simulink model "Powersystem_without_oscilloscopes"  (R2022b)
settings: Solver=ode45  StartTime=0.0  StopTime=25.000000  RelTol=1e-4  AbsTol=1e-5  EnableMultiTasking=on
undefined symbols (not defined in the file or in its folder): v_beta
libraries: simulink x11
(part 2 of 2)

== system Powersystem_without_oscilloscopes/Energylimits ==
  note: Power
  note: Energy
  Pref : Inport
  1-D Lookup Table : Lookup_n-D  NumberOfTableDimensions=1  BreakpointsForDimension1=[0,fracdemax,demax,1000*demax]  Table=[dpmax,dpmax,0,0]  InternalRulePriority=Speed  RndMeth=Simplest
  Constant : Constant  Value=dpmin
  Derivative : Derivative
  Integrator : Integrator
  delimit : Saturate  UpperLimit=demax  LowerLimit=demin
  tail control : simulink/Discontinuities/Saturation Dynamic  OutMin=[]  OutMax=[]  OutDataTypeStr=Inherit: Same as second input  OutDataType=sfix(16)  OutScaling=2^-10  DoSatur=off
  Pout : Outport
  wires:
  Integrator/1 -> delimit/1
  delimit/1 -> 1-D Lookup Table/1, Derivative/1
  Derivative/1 -> Pout/1
  1-D Lookup Table/1 -> tail control/1
  Constant/1 -> tail control/3
  Pref/1 -> tail control/2
  tail control/1 -> Integrator/1

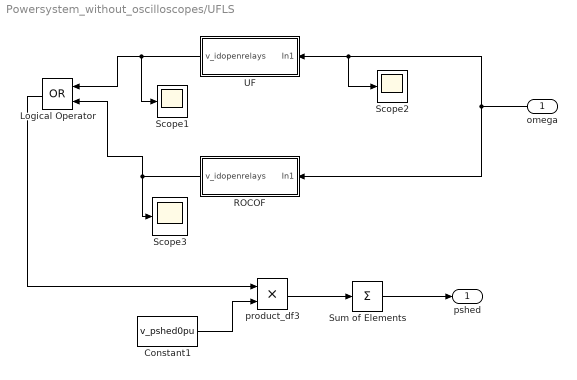
== system Powersystem_without_oscilloscopes/UFLS ==
  omega : Inport
  Constant1 : Constant  Value=v_pshed0pu
  Logical Operator : Logic  Operator=OR  AllPortsSameDT=off  OutDataTypeStr=boolean
  ROCOF : Subsystem
  Scope1 : Scope
  Scope2 : Scope
  Scope3 : Scope
  Sum of Elements : Sum  Inputs=+
  UF : Subsystem
  product_df3 : Product  RndMeth=Zero
  pshed : Outport
  wires:
  omega/1 -> Scope2/1, UF/1(In1), ROCOF/1(In1)
  UF/1(v_idopenrelays) -> Scope1/1, Logical Operator/1
  Sum of Elements/1 -> pshed/1
  Constant1/1 -> product_df3/2
  product_df3/1 -> Sum of Elements/1
  Logical Operator/1 -> product_df3/1
  ROCOF/1(v_idopenrelays) -> Scope3/1, Logical Operator/2

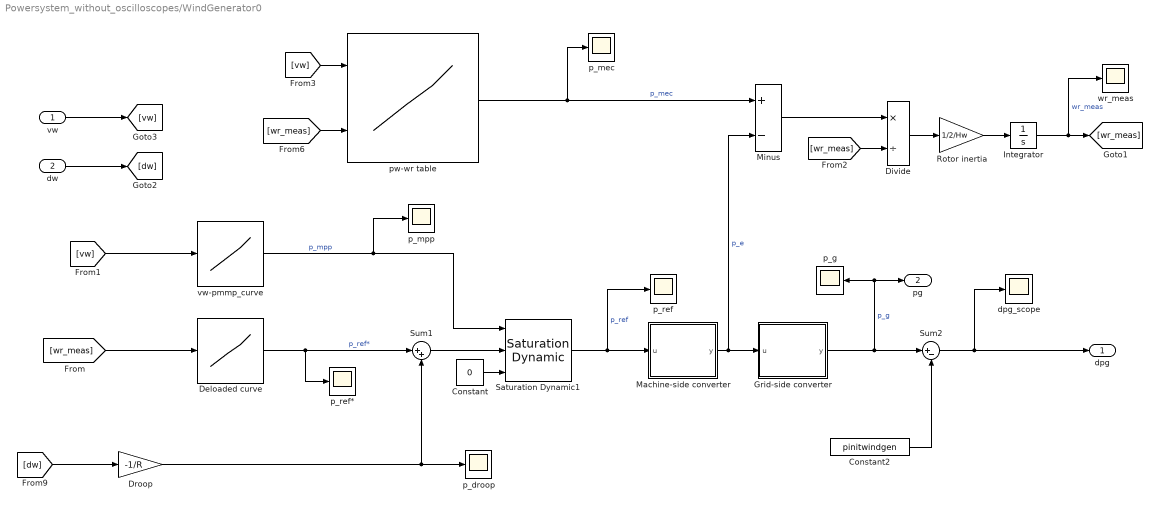
== system Powersystem_without_oscilloscopes/WindGenerator0 ==
  vw : Inport
  dw : Inport  Port=2
  Constant : Constant  Value=0
  Constant2 : Constant  Value=pinitwindgen
  Deloaded curve : Lookup_n-D  NumberOfTableDimensions=1  BreakpointsForDimension1=v_wrdel  Table=v_pwdel  InternalRulePriority=Speed  RndMeth=Simplest
  Divide : Product  Inputs=*/
  Droop : Gain  Gain=-1/R
  Grid-side converter : Subsystem  mask{T=Tc2, y0=pinitwindgen}
      mask prompts: T "Time constant (s)"; y0 "Initial condition (pu)"
  Integrator : Integrator  InitialCondition=wr0
  Machine-side converter : Subsystem  mask{T=Tc1, y0=pinitwindgen}
      mask prompts: T "Time constant (s)"; y0 "Initial condition (pu)"
  Minus : Sum  Inputs=+-
  Rotor inertia : Gain  Gain=1/2/Hw
  Saturation Dynamic1 : simulink/Discontinuities/Saturation Dynamic  OutMin=0  OutMax=[]  OutDataTypeStr=Inherit: Same as second input  OutDataType=fixdt(1, 16)  OutScaling=2^-10  DoSatur=off
  Sum1 : Sum  Inputs=|++
  Sum2 : Sum  Inputs=|+-
  dpg_scope : Scope
  p_droop : Scope
  p_g : Scope
  p_mec : Scope
  p_mpp : Scope
  p_ref : Scope
  p_ref* : Scope
  pw-wr table : Lookup_n-D  BreakpointsForDimension1=v_vw  BreakpointsForDimension2=v_wr  BreakpointsForDimension3=v_beta  Table=m_pw  InternalRulePriority=Speed  RndMeth=Simplest
      settings: InputPortMap=u0,u1
  vw-pmmp_curve : Lookup_n-D  NumberOfTableDimensions=1  BreakpointsForDimension1=v_vw  Table=v_pwmpp  InternalRulePriority=Speed  RndMeth=Simplest
  wr_meas : Scope
  dpg : Outport
  pg : Outport  Port=2
  wires:
  Sum2/1 -> dpg/1, dpg_scope/1
  [wr_meas] -> pw-wr table/2
  Deloaded curve/1 -> Sum1/1, p_ref*/1  "p_ref*"
  [dw] -> Droop/1
  Grid-side converter/1(y) -> Sum2/1, p_g/1, pg/1  "p_g"
  Saturation Dynamic1/1 -> p_ref/1, Machine-side converter/1(u)  "p_ref"
  [wr_meas] -> Deloaded curve/1
  Rotor inertia/1 -> Integrator/1
  [vw] -> pw-wr table/1
  pw-wr table/1 -> Minus/1, p_mec/1  "p_mec"
  Integrator/1 -> wr_meas/1, [wr_meas]  "wr_meas"
  vw/1 -> [vw]
  Sum1/1 -> Saturation Dynamic1/2
  Machine-side converter/1(y) -> Minus/2, Grid-side converter/1(u)  "p_e"
  vw-pmmp_curve/1 -> Saturation Dynamic1/1, p_mpp/1  "p_mpp"
  Constant2/1 -> Sum2/2
  dw/1 -> [dw]
  Constant/1 -> Saturation Dynamic1/3
  [vw] -> vw-pmmp_curve/1
  Droop/1 -> p_droop/1, Sum1/2
  Minus/1 -> Divide/1
  Divide/1 -> Rotor inertia/1
  [wr_meas] -> Divide/2

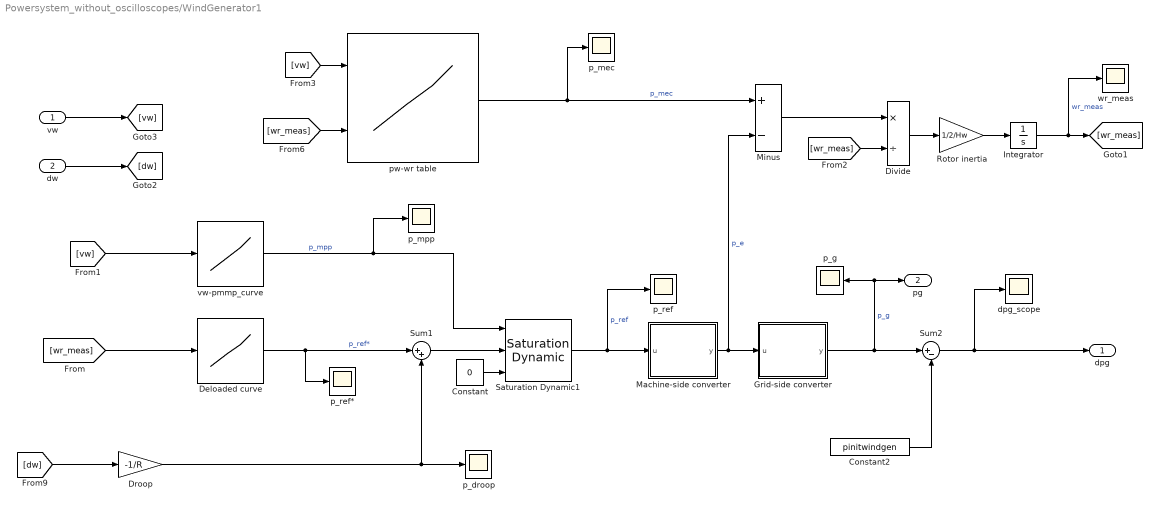
== system Powersystem_without_oscilloscopes/WindGenerator1 ==
  vw : Inport
  dw : Inport  Port=2
  Constant : Constant  Value=0
  Constant2 : Constant  Value=pinitwindgen
  Deloaded curve : Lookup_n-D  NumberOfTableDimensions=1  BreakpointsForDimension1=v_wrdel  Table=v_pwdel  InternalRulePriority=Speed  RndMeth=Simplest
  Divide : Product  Inputs=*/
  Droop : Gain  Gain=-1/R
  Grid-side converter : Subsystem  mask{T=Tc2, y0=pinitwindgen}
      mask prompts: T "Time constant (s)"; y0 "Initial condition (pu)"
  Integrator : Integrator  InitialCondition=wr0
  Machine-side converter : Subsystem  mask{T=Tc1, y0=pinitwindgen}
      mask prompts: T "Time constant (s)"; y0 "Initial condition (pu)"
  Minus : Sum  Inputs=+-
  Rotor inertia : Gain  Gain=1/2/Hw
  Saturation Dynamic1 : simulink/Discontinuities/Saturation Dynamic  OutMin=0  OutMax=[]  OutDataTypeStr=Inherit: Same as second input  OutDataType=fixdt(1, 16)  OutScaling=2^-10  DoSatur=off
  Sum1 : Sum  Inputs=|++
  Sum2 : Sum  Inputs=|+-
  dpg_scope : Scope
  p_droop : Scope
  p_g : Scope
  p_mec : Scope
  p_mpp : Scope
  p_ref : Scope
  p_ref* : Scope
  pw-wr table : Lookup_n-D  BreakpointsForDimension1=v_vw  BreakpointsForDimension2=v_wr  BreakpointsForDimension3=v_beta  Table=m_pw  InternalRulePriority=Speed  RndMeth=Simplest
      settings: InputPortMap=u0,u1
  vw-pmmp_curve : Lookup_n-D  NumberOfTableDimensions=1  BreakpointsForDimension1=v_vw  Table=v_pwmpp  InternalRulePriority=Speed  RndMeth=Simplest
  wr_meas : Scope
  dpg : Outport
  pg : Outport  Port=2
  wires:
  Sum2/1 -> dpg/1, dpg_scope/1
  [wr_meas] -> pw-wr table/2
  Deloaded curve/1 -> Sum1/1, p_ref*/1  "p_ref*"
  [dw] -> Droop/1
  Grid-side converter/1(y) -> Sum2/1, p_g/1, pg/1  "p_g"
  Saturation Dynamic1/1 -> p_ref/1, Machine-side converter/1(u)  "p_ref"
  [wr_meas] -> Deloaded curve/1
  Rotor inertia/1 -> Integrator/1
  [vw] -> pw-wr table/1
  pw-wr table/1 -> Minus/1, p_mec/1  "p_mec"
  Integrator/1 -> wr_meas/1, [wr_meas]  "wr_meas"
  vw/1 -> [vw]
  Sum1/1 -> Saturation Dynamic1/2
  Machine-side converter/1(y) -> Minus/2, Grid-side converter/1(u)  "p_e"
  vw-pmmp_curve/1 -> Saturation Dynamic1/1, p_mpp/1  "p_mpp"
  Constant2/1 -> Sum2/2
  dw/1 -> [dw]
  Constant/1 -> Saturation Dynamic1/3
  [vw] -> vw-pmmp_curve/1
  Droop/1 -> p_droop/1, Sum1/2
  Minus/1 -> Divide/1
  Divide/1 -> Rotor inertia/1
  [wr_meas] -> Divide/2

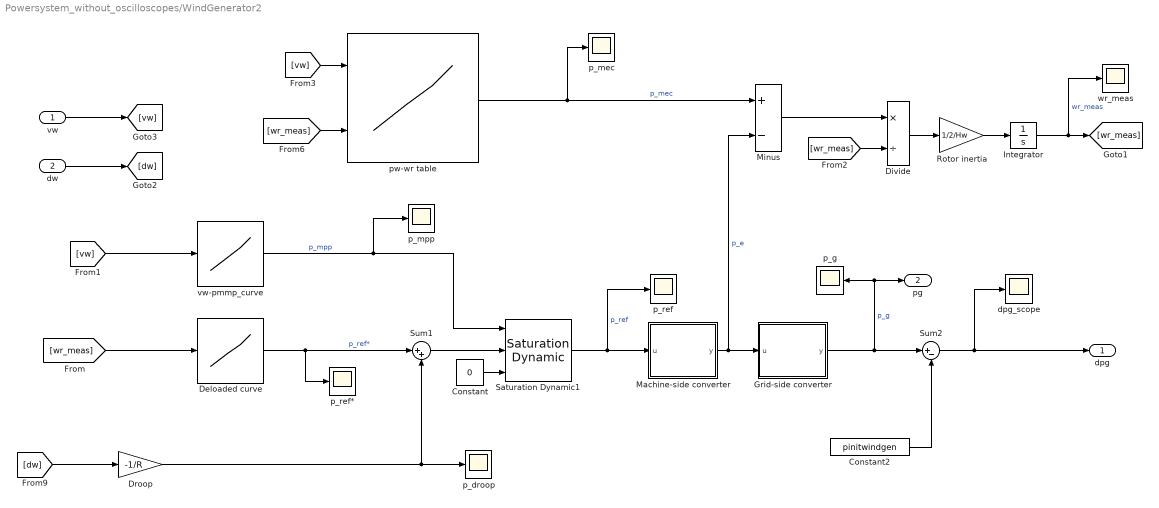
== system Powersystem_without_oscilloscopes/WindGenerator2 ==
  vw : Inport
  dw : Inport  Port=2
  Constant : Constant  Value=0
  Constant2 : Constant  Value=pinitwindgen
  Deloaded curve : Lookup_n-D  NumberOfTableDimensions=1  BreakpointsForDimension1=v_wrdel  Table=v_pwdel  InternalRulePriority=Speed  RndMeth=Simplest
  Divide : Product  Inputs=*/
  Droop : Gain  Gain=-1/R
  Grid-side converter : Subsystem  mask{T=Tc2, y0=pinitwindgen}
      mask prompts: T "Time constant (s)"; y0 "Initial condition (pu)"
  Integrator : Integrator  InitialCondition=wr0
  Machine-side converter : Subsystem  mask{T=Tc1, y0=pinitwindgen}
      mask prompts: T "Time constant (s)"; y0 "Initial condition (pu)"
  Minus : Sum  Inputs=+-
  Rotor inertia : Gain  Gain=1/2/Hw
  Saturation Dynamic1 : simulink/Discontinuities/Saturation Dynamic  OutMin=0  OutMax=[]  OutDataTypeStr=Inherit: Same as second input  OutDataType=fixdt(1, 16)  OutScaling=2^-10  DoSatur=off
  Sum1 : Sum  Inputs=|++
  Sum2 : Sum  Inputs=|+-
  dpg_scope : Scope
  p_droop : Scope
  p_g : Scope
  p_mec : Scope
  p_mpp : Scope
  p_ref : Scope
  p_ref* : Scope
  pw-wr table : Lookup_n-D  BreakpointsForDimension1=v_vw  BreakpointsForDimension2=v_wr  BreakpointsForDimension3=v_beta  Table=m_pw  InternalRulePriority=Speed  RndMeth=Simplest
      settings: InputPortMap=u0,u1
  vw-pmmp_curve : Lookup_n-D  NumberOfTableDimensions=1  BreakpointsForDimension1=v_vw  Table=v_pwmpp  InternalRulePriority=Speed  RndMeth=Simplest
  wr_meas : Scope
  dpg : Outport
  pg : Outport  Port=2
  wires:
  Sum2/1 -> dpg/1, dpg_scope/1
  [wr_meas] -> pw-wr table/2
  Deloaded curve/1 -> Sum1/1, p_ref*/1  "p_ref*"
  [dw] -> Droop/1
  Grid-side converter/1(y) -> Sum2/1, p_g/1, pg/1  "p_g"
  Saturation Dynamic1/1 -> p_ref/1, Machine-side converter/1(u)  "p_ref"
  [wr_meas] -> Deloaded curve/1
  Rotor inertia/1 -> Integrator/1
  [vw] -> pw-wr table/1
  pw-wr table/1 -> Minus/1, p_mec/1  "p_mec"
  Integrator/1 -> wr_meas/1, [wr_meas]  "wr_meas"
  vw/1 -> [vw]
  Sum1/1 -> Saturation Dynamic1/2
  Machine-side converter/1(y) -> Minus/2, Grid-side converter/1(u)  "p_e"
  vw-pmmp_curve/1 -> Saturation Dynamic1/1, p_mpp/1  "p_mpp"
  Constant2/1 -> Sum2/2
  dw/1 -> [dw]
  Constant/1 -> Saturation Dynamic1/3
  [vw] -> vw-pmmp_curve/1
  Droop/1 -> p_droop/1, Sum1/2
  Minus/1 -> Divide/1
  Divide/1 -> Rotor inertia/1
  [wr_meas] -> Divide/2

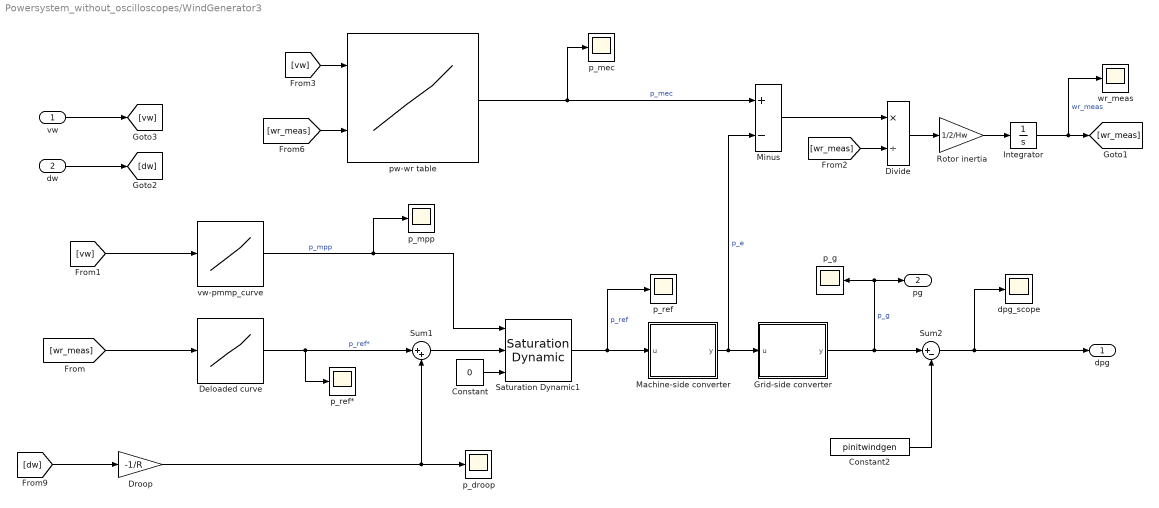
== system Powersystem_without_oscilloscopes/WindGenerator3 ==
  vw : Inport
  dw : Inport  Port=2
  Constant : Constant  Value=0
  Constant2 : Constant  Value=pinitwindgen
  Deloaded curve : Lookup_n-D  NumberOfTableDimensions=1  BreakpointsForDimension1=v_wrdel  Table=v_pwdel  InternalRulePriority=Speed  RndMeth=Simplest
  Divide : Product  Inputs=*/
  Droop : Gain  Gain=-1/R
  Grid-side converter : Subsystem  mask{T=Tc2, y0=pinitwindgen}
      mask prompts: T "Time constant (s)"; y0 "Initial condition (pu)"
  Integrator : Integrator  InitialCondition=wr0
  Machine-side converter : Subsystem  mask{T=Tc1, y0=pinitwindgen}
      mask prompts: T "Time constant (s)"; y0 "Initial condition (pu)"
  Minus : Sum  Inputs=+-
  Rotor inertia : Gain  Gain=1/2/Hw
  Saturation Dynamic1 : simulink/Discontinuities/Saturation Dynamic  OutMin=0  OutMax=[]  OutDataTypeStr=Inherit: Same as second input  OutDataType=fixdt(1, 16)  OutScaling=2^-10  DoSatur=off
  Sum1 : Sum  Inputs=|++
  Sum2 : Sum  Inputs=|+-
  dpg_scope : Scope
  p_droop : Scope
  p_g : Scope
  p_mec : Scope
  p_mpp : Scope
  p_ref : Scope
  p_ref* : Scope
  pw-wr table : Lookup_n-D  BreakpointsForDimension1=v_vw  BreakpointsForDimension2=v_wr  BreakpointsForDimension3=v_beta  Table=m_pw  InternalRulePriority=Speed  RndMeth=Simplest
      settings: InputPortMap=u0,u1
  vw-pmmp_curve : Lookup_n-D  NumberOfTableDimensions=1  BreakpointsForDimension1=v_vw  Table=v_pwmpp  InternalRulePriority=Speed  RndMeth=Simplest
  wr_meas : Scope
  dpg : Outport
  pg : Outport  Port=2
  wires:
  Sum2/1 -> dpg/1, dpg_scope/1
  [wr_meas] -> pw-wr table/2
  Deloaded curve/1 -> Sum1/1, p_ref*/1  "p_ref*"
  [dw] -> Droop/1
  Grid-side converter/1(y) -> Sum2/1, p_g/1, pg/1  "p_g"
  Saturation Dynamic1/1 -> p_ref/1, Machine-side converter/1(u)  "p_ref"
  [wr_meas] -> Deloaded curve/1
  Rotor inertia/1 -> Integrator/1
  [vw] -> pw-wr table/1
  pw-wr table/1 -> Minus/1, p_mec/1  "p_mec"
  Integrator/1 -> wr_meas/1, [wr_meas]  "wr_meas"
  vw/1 -> [vw]
  Sum1/1 -> Saturation Dynamic1/2
  Machine-side converter/1(y) -> Minus/2, Grid-side converter/1(u)  "p_e"
  vw-pmmp_curve/1 -> Saturation Dynamic1/1, p_mpp/1  "p_mpp"
  Constant2/1 -> Sum2/2
  dw/1 -> [dw]
  Constant/1 -> Saturation Dynamic1/3
  [vw] -> vw-pmmp_curve/1
  Droop/1 -> p_droop/1, Sum1/2
  Minus/1 -> Divide/1
  Divide/1 -> Rotor inertia/1
  [wr_meas] -> Divide/2

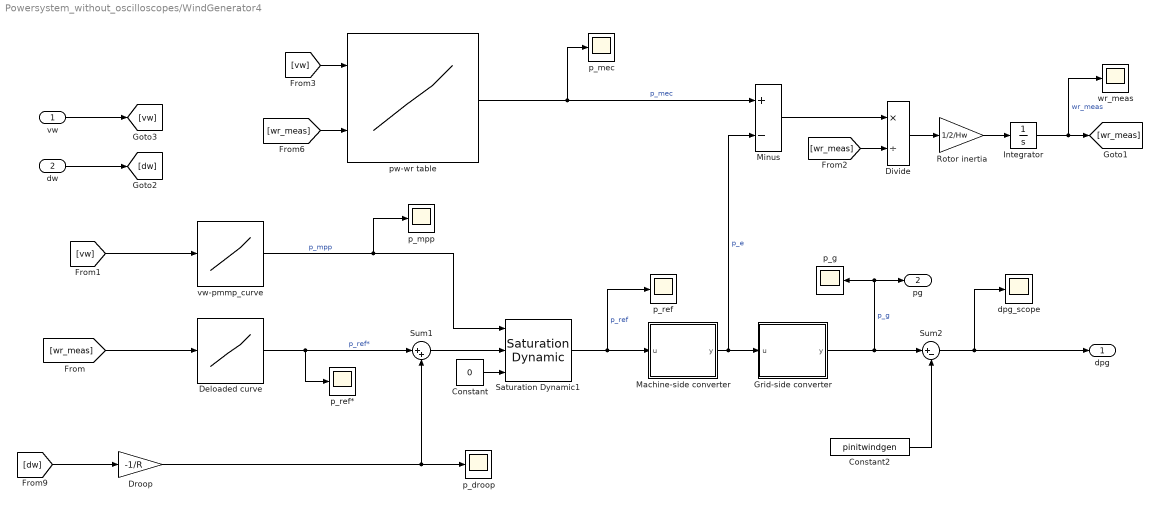
== system Powersystem_without_oscilloscopes/WindGenerator4 ==
  vw : Inport
  dw : Inport  Port=2
  Constant : Constant  Value=0
  Constant2 : Constant  Value=pinitwindgen
  Deloaded curve : Lookup_n-D  NumberOfTableDimensions=1  BreakpointsForDimension1=v_wrdel  Table=v_pwdel  InternalRulePriority=Speed  RndMeth=Simplest
  Divide : Product  Inputs=*/
  Droop : Gain  Gain=-1/R
  Grid-side converter : Subsystem  mask{T=Tc2, y0=pinitwindgen}
      mask prompts: T "Time constant (s)"; y0 "Initial condition (pu)"
  Integrator : Integrator  InitialCondition=wr0
  Machine-side converter : Subsystem  mask{T=Tc1, y0=pinitwindgen}
      mask prompts: T "Time constant (s)"; y0 "Initial condition (pu)"
  Minus : Sum  Inputs=+-
  Rotor inertia : Gain  Gain=1/2/Hw
  Saturation Dynamic1 : simulink/Discontinuities/Saturation Dynamic  OutMin=0  OutMax=[]  OutDataTypeStr=Inherit: Same as second input  OutDataType=fixdt(1, 16)  OutScaling=2^-10  DoSatur=off
  Sum1 : Sum  Inputs=|++
  Sum2 : Sum  Inputs=|+-
  dpg_scope : Scope
  p_droop : Scope
  p_g : Scope
  p_mec : Scope
  p_mpp : Scope
  p_ref : Scope
  p_ref* : Scope
  pw-wr table : Lookup_n-D  BreakpointsForDimension1=v_vw  BreakpointsForDimension2=v_wr  BreakpointsForDimension3=v_beta  Table=m_pw  InternalRulePriority=Speed  RndMeth=Simplest
      settings: InputPortMap=u0,u1
  vw-pmmp_curve : Lookup_n-D  NumberOfTableDimensions=1  BreakpointsForDimension1=v_vw  Table=v_pwmpp  InternalRulePriority=Speed  RndMeth=Simplest
  wr_meas : Scope
  dpg : Outport
  pg : Outport  Port=2
  wires:
  Sum2/1 -> dpg/1, dpg_scope/1
  [wr_meas] -> pw-wr table/2
  Deloaded curve/1 -> Sum1/1, p_ref*/1  "p_ref*"
  [dw] -> Droop/1
  Grid-side converter/1(y) -> Sum2/1, p_g/1, pg/1  "p_g"
  Saturation Dynamic1/1 -> p_ref/1, Machine-side converter/1(u)  "p_ref"
  [wr_meas] -> Deloaded curve/1
  Rotor inertia/1 -> Integrator/1
  [vw] -> pw-wr table/1
  pw-wr table/1 -> Minus/1, p_mec/1  "p_mec"
  Integrator/1 -> wr_meas/1, [wr_meas]  "wr_meas"
  vw/1 -> [vw]
  Sum1/1 -> Saturation Dynamic1/2
  Machine-side converter/1(y) -> Minus/2, Grid-side converter/1(u)  "p_e"
  vw-pmmp_curve/1 -> Saturation Dynamic1/1, p_mpp/1  "p_mpp"
  Constant2/1 -> Sum2/2
  dw/1 -> [dw]
  Constant/1 -> Saturation Dynamic1/3
  [vw] -> vw-pmmp_curve/1
  Droop/1 -> p_droop/1, Sum1/2
  Minus/1 -> Divide/1
  Divide/1 -> Rotor inertia/1
  [wr_meas] -> Divide/2

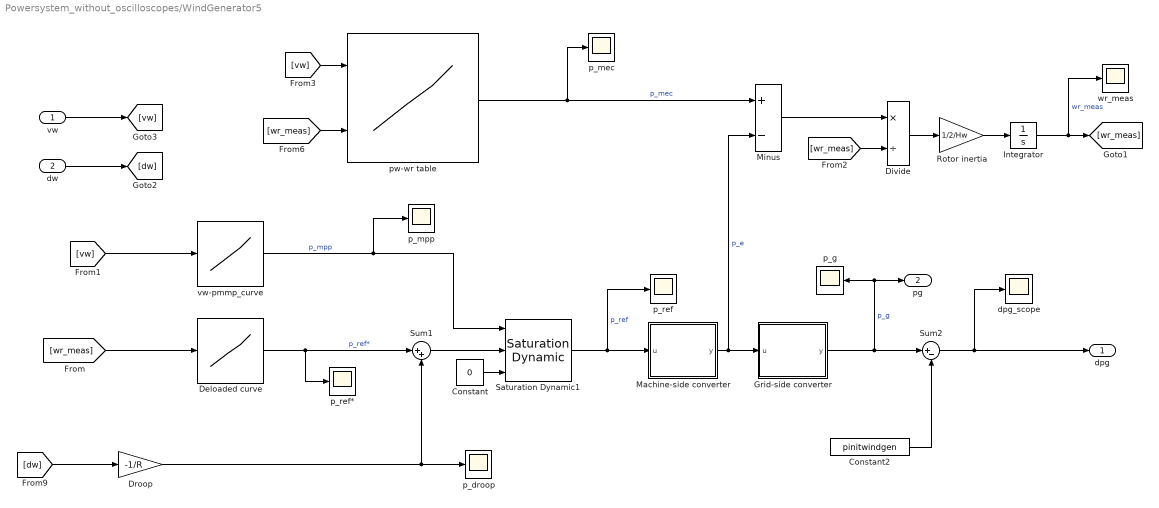
== system Powersystem_without_oscilloscopes/WindGenerator5 ==
  vw : Inport
  dw : Inport  Port=2
  Constant : Constant  Value=0
  Constant2 : Constant  Value=pinitwindgen
  Deloaded curve : Lookup_n-D  NumberOfTableDimensions=1  BreakpointsForDimension1=v_wrdel  Table=v_pwdel  InternalRulePriority=Speed  RndMeth=Simplest
  Divide : Product  Inputs=*/
  Droop : Gain  Gain=-1/R
  Grid-side converter : Subsystem  mask{T=Tc2, y0=pinitwindgen}
      mask prompts: T "Time constant (s)"; y0 "Initial condition (pu)"
  Integrator : Integrator  InitialCondition=wr0
  Machine-side converter : Subsystem  mask{T=Tc1, y0=pinitwindgen}
      mask prompts: T "Time constant (s)"; y0 "Initial condition (pu)"
  Minus : Sum  Inputs=+-
  Rotor inertia : Gain  Gain=1/2/Hw
  Saturation Dynamic1 : simulink/Discontinuities/Saturation Dynamic  OutMin=0  OutMax=[]  OutDataTypeStr=Inherit: Same as second input  OutDataType=fixdt(1, 16)  OutScaling=2^-10  DoSatur=off
  Sum1 : Sum  Inputs=|++
  Sum2 : Sum  Inputs=|+-
  dpg_scope : Scope
  p_droop : Scope
  p_g : Scope
  p_mec : Scope
  p_mpp : Scope
  p_ref : Scope
  p_ref* : Scope
  pw-wr table : Lookup_n-D  BreakpointsForDimension1=v_vw  BreakpointsForDimension2=v_wr  BreakpointsForDimension3=v_beta  Table=m_pw  InternalRulePriority=Speed  RndMeth=Simplest
      settings: InputPortMap=u0,u1
  vw-pmmp_curve : Lookup_n-D  NumberOfTableDimensions=1  BreakpointsForDimension1=v_vw  Table=v_pwmpp  InternalRulePriority=Speed  RndMeth=Simplest
  wr_meas : Scope
  dpg : Outport
  pg : Outport  Port=2
  wires:
  Sum2/1 -> dpg/1, dpg_scope/1
  [wr_meas] -> pw-wr table/2
  Deloaded curve/1 -> Sum1/1, p_ref*/1  "p_ref*"
  [dw] -> Droop/1
  Grid-side converter/1(y) -> Sum2/1, p_g/1, pg/1  "p_g"
  Saturation Dynamic1/1 -> p_ref/1, Machine-side converter/1(u)  "p_ref"
  [wr_meas] -> Deloaded curve/1
  Rotor inertia/1 -> Integrator/1
  [vw] -> pw-wr table/1
  pw-wr table/1 -> Minus/1, p_mec/1  "p_mec"
  Integrator/1 -> wr_meas/1, [wr_meas]  "wr_meas"
  vw/1 -> [vw]
  Sum1/1 -> Saturation Dynamic1/2
  Machine-side converter/1(y) -> Minus/2, Grid-side converter/1(u)  "p_e"
  vw-pmmp_curve/1 -> Saturation Dynamic1/1, p_mpp/1  "p_mpp"
  Constant2/1 -> Sum2/2
  dw/1 -> [dw]
  Constant/1 -> Saturation Dynamic1/3
  [vw] -> vw-pmmp_curve/1
  Droop/1 -> p_droop/1, Sum1/2
  Minus/1 -> Divide/1
  Divide/1 -> Rotor inertia/1
  [wr_meas] -> Divide/2

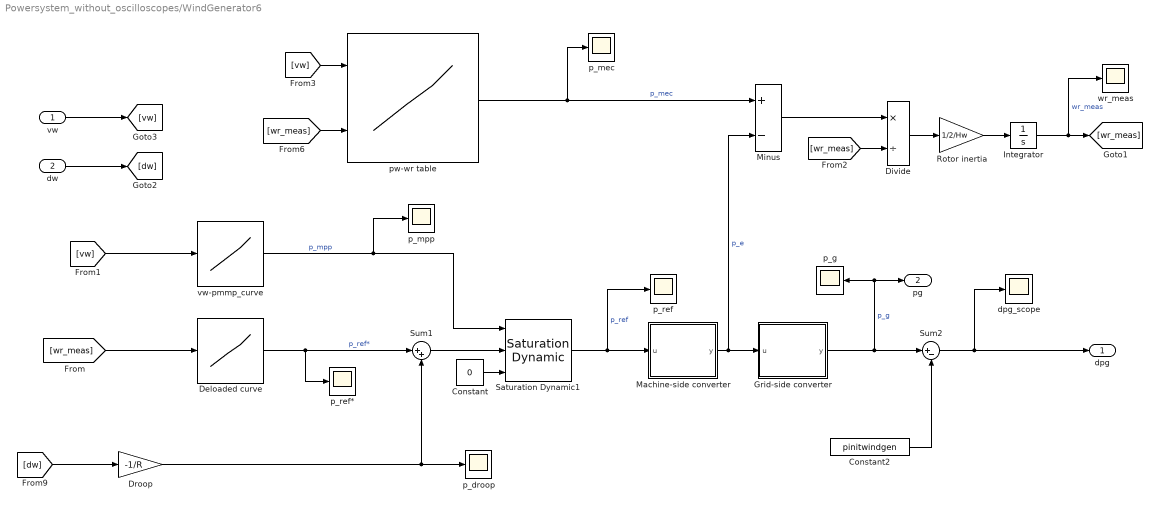
== system Powersystem_without_oscilloscopes/WindGenerator6 ==
  vw : Inport
  dw : Inport  Port=2
  Constant : Constant  Value=0
  Constant2 : Constant  Value=pinitwindgen
  Deloaded curve : Lookup_n-D  NumberOfTableDimensions=1  BreakpointsForDimension1=v_wrdel  Table=v_pwdel  InternalRulePriority=Speed  RndMeth=Simplest
  Divide : Product  Inputs=*/
  Droop : Gain  Gain=-1/R
  Grid-side converter : Subsystem  mask{T=Tc2, y0=pinitwindgen}
      mask prompts: T "Time constant (s)"; y0 "Initial condition (pu)"
  Integrator : Integrator  InitialCondition=wr0
  Machine-side converter : Subsystem  mask{T=Tc1, y0=pinitwindgen}
      mask prompts: T "Time constant (s)"; y0 "Initial condition (pu)"
  Minus : Sum  Inputs=+-
  Rotor inertia : Gain  Gain=1/2/Hw
  Saturation Dynamic1 : simulink/Discontinuities/Saturation Dynamic  OutMin=0  OutMax=[]  OutDataTypeStr=Inherit: Same as second input  OutDataType=fixdt(1, 16)  OutScaling=2^-10  DoSatur=off
  Sum1 : Sum  Inputs=|++
  Sum2 : Sum  Inputs=|+-
  dpg_scope : Scope
  p_droop : Scope
  p_g : Scope
  p_mec : Scope
  p_mpp : Scope
  p_ref : Scope
  p_ref* : Scope
  pw-wr table : Lookup_n-D  BreakpointsForDimension1=v_vw  BreakpointsForDimension2=v_wr  BreakpointsForDimension3=v_beta  Table=m_pw  InternalRulePriority=Speed  RndMeth=Simplest
      settings: InputPortMap=u0,u1
  vw-pmmp_curve : Lookup_n-D  NumberOfTableDimensions=1  BreakpointsForDimension1=v_vw  Table=v_pwmpp  InternalRulePriority=Speed  RndMeth=Simplest
  wr_meas : Scope
  dpg : Outport
  pg : Outport  Port=2
  wires:
  Sum2/1 -> dpg/1, dpg_scope/1
  [wr_meas] -> pw-wr table/2
  Deloaded curve/1 -> Sum1/1, p_ref*/1  "p_ref*"
  [dw] -> Droop/1
  Grid-side converter/1(y) -> Sum2/1, p_g/1, pg/1  "p_g"
  Saturation Dynamic1/1 -> p_ref/1, Machine-side converter/1(u)  "p_ref"
  [wr_meas] -> Deloaded curve/1
  Rotor inertia/1 -> Integrator/1
  [vw] -> pw-wr table/1
  pw-wr table/1 -> Minus/1, p_mec/1  "p_mec"
  Integrator/1 -> wr_meas/1, [wr_meas]  "wr_meas"
  vw/1 -> [vw]
  Sum1/1 -> Saturation Dynamic1/2
  Machine-side converter/1(y) -> Minus/2, Grid-side converter/1(u)  "p_e"
  vw-pmmp_curve/1 -> Saturation Dynamic1/1, p_mpp/1  "p_mpp"
  Constant2/1 -> Sum2/2
  dw/1 -> [dw]
  Constant/1 -> Saturation Dynamic1/3
  [vw] -> vw-pmmp_curve/1
  Droop/1 -> p_droop/1, Sum1/2
  Minus/1 -> Divide/1
  Divide/1 -> Rotor inertia/1
  [wr_meas] -> Divide/2

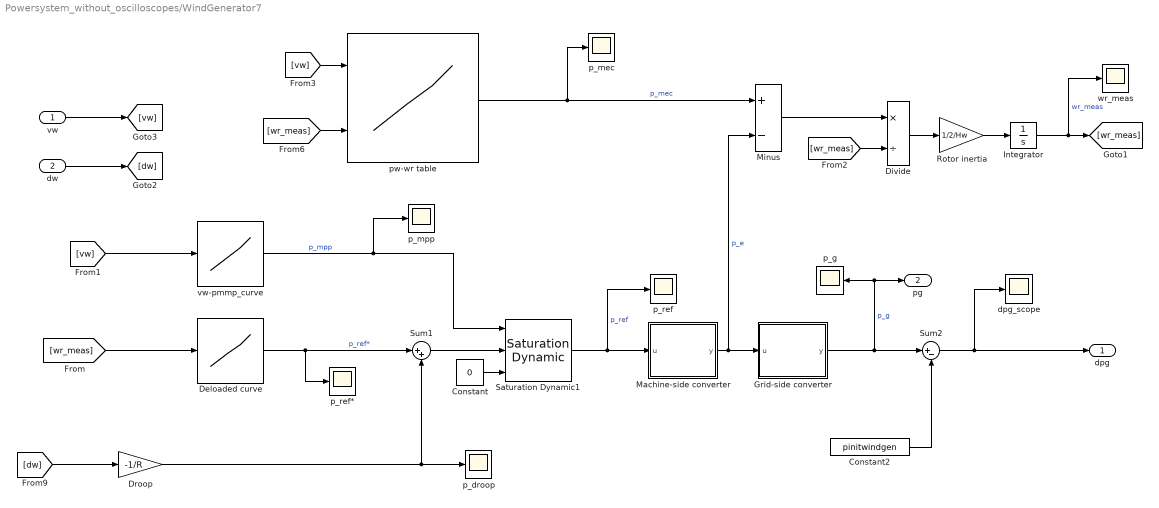
== system Powersystem_without_oscilloscopes/WindGenerator7 ==
  vw : Inport
  dw : Inport  Port=2
  Constant : Constant  Value=0
  Constant2 : Constant  Value=pinitwindgen
  Deloaded curve : Lookup_n-D  NumberOfTableDimensions=1  BreakpointsForDimension1=v_wrdel  Table=v_pwdel  InternalRulePriority=Speed  RndMeth=Simplest
  Divide : Product  Inputs=*/
  Droop : Gain  Gain=-1/R
  Grid-side converter : Subsystem  mask{T=Tc2, y0=pinitwindgen}
      mask prompts: T "Time constant (s)"; y0 "Initial condition (pu)"
  Integrator : Integrator  InitialCondition=wr0
  Machine-side converter : Subsystem  mask{T=Tc1, y0=pinitwindgen}
      mask prompts: T "Time constant (s)"; y0 "Initial condition (pu)"
  Minus : Sum  Inputs=+-
  Rotor inertia : Gain  Gain=1/2/Hw
  Saturation Dynamic1 : simulink/Discontinuities/Saturation Dynamic  OutMin=0  OutMax=[]  OutDataTypeStr=Inherit: Same as second input  OutDataType=fixdt(1, 16)  OutScaling=2^-10  DoSatur=off
  Sum1 : Sum  Inputs=|++
  Sum2 : Sum  Inputs=|+-
  dpg_scope : Scope
  p_droop : Scope
  p_g : Scope
  p_mec : Scope
  p_mpp : Scope
  p_ref : Scope
  p_ref* : Scope
  pw-wr table : Lookup_n-D  BreakpointsForDimension1=v_vw  BreakpointsForDimension2=v_wr  BreakpointsForDimension3=v_beta  Table=m_pw  InternalRulePriority=Speed  RndMeth=Simplest
      settings: InputPortMap=u0,u1
  vw-pmmp_curve : Lookup_n-D  NumberOfTableDimensions=1  BreakpointsForDimension1=v_vw  Table=v_pwmpp  InternalRulePriority=Speed  RndMeth=Simplest
  wr_meas : Scope
  dpg : Outport
  pg : Outport  Port=2
  wires:
  Sum2/1 -> dpg/1, dpg_scope/1
  [wr_meas] -> pw-wr table/2
  Deloaded curve/1 -> Sum1/1, p_ref*/1  "p_ref*"
  [dw] -> Droop/1
  Grid-side converter/1(y) -> Sum2/1, p_g/1, pg/1  "p_g"
  Saturation Dynamic1/1 -> p_ref/1, Machine-side converter/1(u)  "p_ref"
  [wr_meas] -> Deloaded curve/1
  Rotor inertia/1 -> Integrator/1
  [vw] -> pw-wr table/1
  pw-wr table/1 -> Minus/1, p_mec/1  "p_mec"
  Integrator/1 -> wr_meas/1, [wr_meas]  "wr_meas"
  vw/1 -> [vw]
  Sum1/1 -> Saturation Dynamic1/2
  Machine-side converter/1(y) -> Minus/2, Grid-side converter/1(u)  "p_e"
  vw-pmmp_curve/1 -> Saturation Dynamic1/1, p_mpp/1  "p_mpp"
  Constant2/1 -> Sum2/2
  dw/1 -> [dw]
  Constant/1 -> Saturation Dynamic1/3
  [vw] -> vw-pmmp_curve/1
  Droop/1 -> p_droop/1, Sum1/2
  Minus/1 -> Divide/1
  Divide/1 -> Rotor inertia/1
  [wr_meas] -> Divide/2

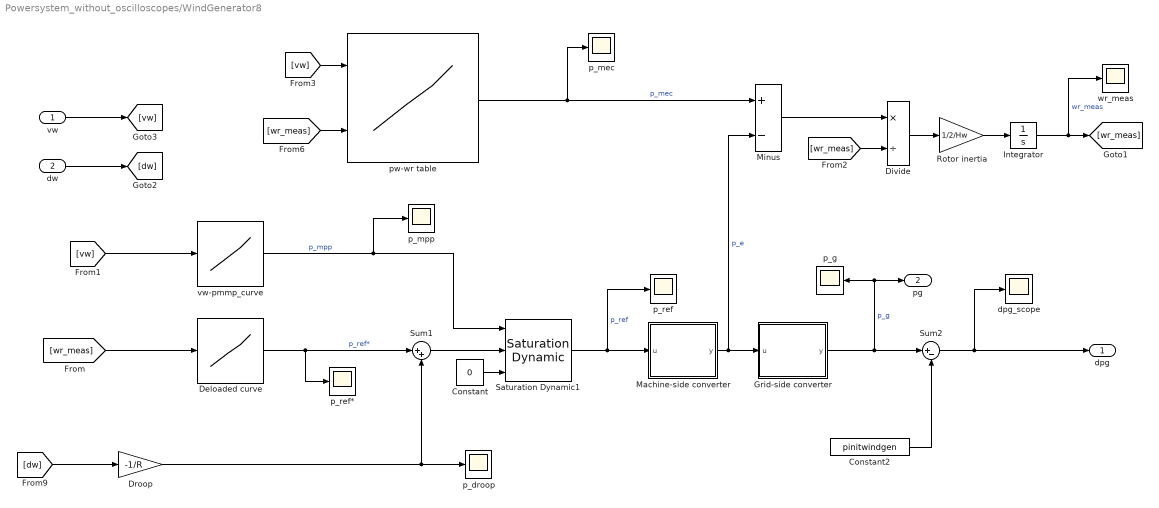
== system Powersystem_without_oscilloscopes/WindGenerator8 ==
  vw : Inport
  dw : Inport  Port=2
  Constant : Constant  Value=0
  Constant2 : Constant  Value=pinitwindgen
  Deloaded curve : Lookup_n-D  NumberOfTableDimensions=1  BreakpointsForDimension1=v_wrdel  Table=v_pwdel  InternalRulePriority=Speed  RndMeth=Simplest
  Divide : Product  Inputs=*/
  Droop : Gain  Gain=-1/R
  Grid-side converter : Subsystem  mask{T=Tc2, y0=pinitwindgen}
      mask prompts: T "Time constant (s)"; y0 "Initial condition (pu)"
  Integrator : Integrator  InitialCondition=wr0
  Machine-side converter : Subsystem  mask{T=Tc1, y0=pinitwindgen}
      mask prompts: T "Time constant (s)"; y0 "Initial condition (pu)"
  Minus : Sum  Inputs=+-
  Rotor inertia : Gain  Gain=1/2/Hw
  Saturation Dynamic1 : simulink/Discontinuities/Saturation Dynamic  OutMin=0  OutMax=[]  OutDataTypeStr=Inherit: Same as second input  OutDataType=fixdt(1, 16)  OutScaling=2^-10  DoSatur=off
  Sum1 : Sum  Inputs=|++
  Sum2 : Sum  Inputs=|+-
  dpg_scope : Scope
  p_droop : Scope
  p_g : Scope
  p_mec : Scope
  p_mpp : Scope
  p_ref : Scope
  p_ref* : Scope
  pw-wr table : Lookup_n-D  BreakpointsForDimension1=v_vw  BreakpointsForDimension2=v_wr  BreakpointsForDimension3=v_beta  Table=m_pw  InternalRulePriority=Speed  RndMeth=Simplest
      settings: InputPortMap=u0,u1
  vw-pmmp_curve : Lookup_n-D  NumberOfTableDimensions=1  BreakpointsForDimension1=v_vw  Table=v_pwmpp  InternalRulePriority=Speed  RndMeth=Simplest
  wr_meas : Scope
  dpg : Outport
  pg : Outport  Port=2
  wires:
  Sum2/1 -> dpg/1, dpg_scope/1
  [wr_meas] -> pw-wr table/2
  Deloaded curve/1 -> Sum1/1, p_ref*/1  "p_ref*"
  [dw] -> Droop/1
  Grid-side converter/1(y) -> Sum2/1, p_g/1, pg/1  "p_g"
  Saturation Dynamic1/1 -> p_ref/1, Machine-side converter/1(u)  "p_ref"
  [wr_meas] -> Deloaded curve/1
  Rotor inertia/1 -> Integrator/1
  [vw] -> pw-wr table/1
  pw-wr table/1 -> Minus/1, p_mec/1  "p_mec"
  Integrator/1 -> wr_meas/1, [wr_meas]  "wr_meas"
  vw/1 -> [vw]
  Sum1/1 -> Saturation Dynamic1/2
  Machine-side converter/1(y) -> Minus/2, Grid-side converter/1(u)  "p_e"
  vw-pmmp_curve/1 -> Saturation Dynamic1/1, p_mpp/1  "p_mpp"
  Constant2/1 -> Sum2/2
  dw/1 -> [dw]
  Constant/1 -> Saturation Dynamic1/3
  [vw] -> vw-pmmp_curve/1
  Droop/1 -> p_droop/1, Sum1/2
  Minus/1 -> Divide/1
  Divide/1 -> Rotor inertia/1
  [wr_meas] -> Divide/2

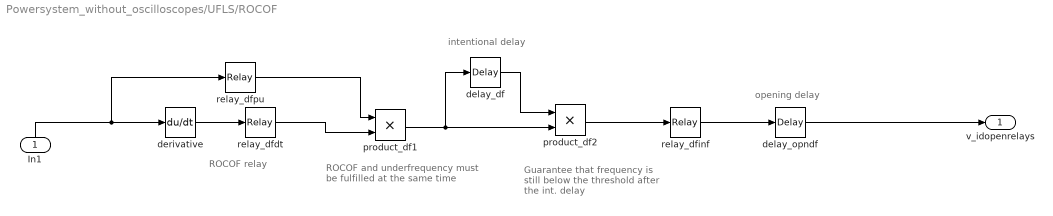
== system Powersystem_without_oscilloscopes/UFLS/ROCOF ==
  note: Guarantee that frequency
      | is still below the threshold
      | after the int. delay
  note: ROCOF relay
  note: ROCOF and underfrequency
      | must be fulfilled at the same time
  note: intentional delay
  note: opening delay
  In1 : Inport
  delay_df : TransportDelay  DelayTime=v_tintrocof
  delay_opndf : TransportDelay  DelayTime=v_topnrocof
  derivative : Derivative
  product_df1 : Product  RndMeth=Zero
  product_df2 : Product  RndMeth=Zero
  relay_dfdt : Relay  OnSwitchValue=v_dfdtrocofpu  OffSwitchValue=v_dfdtrocofpu  OnOutputValue=0  OffOutputValue=1
  relay_dfinf : Relay  OnSwitchValue=1  OffSwitchValue=-1
  relay_dfpu : Relay  OnSwitchValue=v_dfrocofpu  OffSwitchValue=v_dfrocofpu  OnOutputValue=0  OffOutputValue=1
  v_idopenrelays : Outport
  wires:
  In1/1 -> relay_dfpu/1, derivative/1
  relay_dfdt/1 -> product_df1/2
  delay_opndf/1 -> v_idopenrelays/1
  relay_dfinf/1 -> delay_opndf/1
  product_df2/1 -> relay_dfinf/1
  delay_df/1 -> product_df2/1
  product_df1/1 -> product_df2/2, delay_df/1
  derivative/1 -> relay_dfdt/1
  relay_dfpu/1 -> product_df1/1

== system Powersystem_without_oscilloscopes/UFLS/UF ==
  note: Guarantee that frequency
      | is still below the threshold
      | after the int. delay
  note: ROCOF relay
  note: ROCOF and underfrequency
      | must be fulfilled at the same time
  note: intentional delay
  note: opening delay
  In1 : Inport
  delay_df : TransportDelay  DelayTime=v_tintuf
  delay_opndf : TransportDelay  DelayTime=v_topnuf
  derivative : Derivative
  product_df1 : Product  RndMeth=Zero
  product_df2 : Product  RndMeth=Zero
  relay_dfdt : Relay  OnSwitchValue=v_dfdtufpu  OffSwitchValue=v_dfdtufpu  OnOutputValue=0  OffOutputValue=1
  relay_dfinf : Relay  OnSwitchValue=1  OffSwitchValue=-1
  relay_dfpu : Relay  OnSwitchValue=v_dfufpu  OffSwitchValue=v_dfufpu  OnOutputValue=0  OffOutputValue=1
  v_idopenrelays : Outport
  wires:
  In1/1 -> relay_dfpu/1, derivative/1
  relay_dfdt/1 -> product_df1/2
  delay_opndf/1 -> v_idopenrelays/1
  product_df2/1 -> relay_dfinf/1
  delay_df/1 -> product_df2/1
  product_df1/1 -> product_df2/2, delay_df/1
  derivative/1 -> relay_dfdt/1
  relay_dfpu/1 -> product_df1/1
  relay_dfinf/1 -> delay_opndf/1

== system Powersystem_without_oscilloscopes/WindGenerator0/Grid-side converter ==
  u : Inport
  Converter2 : Gain  Gain=1/T
  Integrator2 : Integrator  InitialCondition=y0
  Sum3 : Sum  Inputs=|+-
  y : Outport
  wires:
  Integrator2/1 -> y/1, Sum3/2
  Sum3/1 -> Converter2/1
  Converter2/1 -> Integrator2/1
  u/1 -> Sum3/1

== system Powersystem_without_oscilloscopes/WindGenerator0/Machine-side converter ==
  u : Inport
  Converter2 : Gain  Gain=1/T
  Integrator2 : Integrator  InitialCondition=y0
  Sum3 : Sum  Inputs=|+-
  y : Outport
  wires:
  Integrator2/1 -> y/1, Sum3/2
  Sum3/1 -> Converter2/1
  Converter2/1 -> Integrator2/1
  u/1 -> Sum3/1

== system Powersystem_without_oscilloscopes/WindGenerator1/Grid-side converter ==
  u : Inport
  Converter2 : Gain  Gain=1/T
  Integrator2 : Integrator  InitialCondition=y0
  Sum3 : Sum  Inputs=|+-
  y : Outport
  wires:
  Integrator2/1 -> y/1, Sum3/2
  Sum3/1 -> Converter2/1
  Converter2/1 -> Integrator2/1
  u/1 -> Sum3/1

== system Powersystem_without_oscilloscopes/WindGenerator1/Machine-side converter ==
  u : Inport
  Converter2 : Gain  Gain=1/T
  Integrator2 : Integrator  InitialCondition=y0
  Sum3 : Sum  Inputs=|+-
  y : Outport
  wires:
  Integrator2/1 -> y/1, Sum3/2
  Sum3/1 -> Converter2/1
  Converter2/1 -> Integrator2/1
  u/1 -> Sum3/1

== system Powersystem_without_oscilloscopes/WindGenerator2/Grid-side converter ==
  u : Inport
  Converter2 : Gain  Gain=1/T
  Integrator2 : Integrator  InitialCondition=y0
  Sum3 : Sum  Inputs=|+-
  y : Outport
  wires:
  Integrator2/1 -> y/1, Sum3/2
  Sum3/1 -> Converter2/1
  Converter2/1 -> Integrator2/1
  u/1 -> Sum3/1

== system Powersystem_without_oscilloscopes/WindGenerator2/Machine-side converter ==
  u : Inport
  Converter2 : Gain  Gain=1/T
  Integrator2 : Integrator  InitialCondition=y0
  Sum3 : Sum  Inputs=|+-
  y : Outport
  wires:
  Integrator2/1 -> y/1, Sum3/2
  Sum3/1 -> Converter2/1
  Converter2/1 -> Integrator2/1
  u/1 -> Sum3/1

== system Powersystem_without_oscilloscopes/WindGenerator3/Grid-side converter ==
  u : Inport
  Converter2 : Gain  Gain=1/T
  Integrator2 : Integrator  InitialCondition=y0
  Sum3 : Sum  Inputs=|+-
  y : Outport
  wires:
  Integrator2/1 -> y/1, Sum3/2
  Sum3/1 -> Converter2/1
  Converter2/1 -> Integrator2/1
  u/1 -> Sum3/1

== system Powersystem_without_oscilloscopes/WindGenerator3/Machine-side converter ==
  u : Inport
  Converter2 : Gain  Gain=1/T
  Integrator2 : Integrator  InitialCondition=y0
  Sum3 : Sum  Inputs=|+-
  y : Outport
  wires:
  Integrator2/1 -> y/1, Sum3/2
  Sum3/1 -> Converter2/1
  Converter2/1 -> Integrator2/1
  u/1 -> Sum3/1

== system Powersystem_without_oscilloscopes/WindGenerator4/Grid-side converter ==
  u : Inport
  Converter2 : Gain  Gain=1/T
  Integrator2 : Integrator  InitialCondition=y0
  Sum3 : Sum  Inputs=|+-
  y : Outport
  wires:
  Integrator2/1 -> y/1, Sum3/2
  Sum3/1 -> Converter2/1
  Converter2/1 -> Integrator2/1
  u/1 -> Sum3/1

== system Powersystem_without_oscilloscopes/WindGenerator4/Machine-side converter ==
  u : Inport
  Converter2 : Gain  Gain=1/T
  Integrator2 : Integrator  InitialCondition=y0
  Sum3 : Sum  Inputs=|+-
  y : Outport
  wires:
  Integrator2/1 -> y/1, Sum3/2
  Sum3/1 -> Converter2/1
  Converter2/1 -> Integrator2/1
  u/1 -> Sum3/1

== system Powersystem_without_oscilloscopes/WindGenerator5/Grid-side converter ==
  u : Inport
  Converter2 : Gain  Gain=1/T
  Integrator2 : Integrator  InitialCondition=y0
  Sum3 : Sum  Inputs=|+-
  y : Outport
  wires:
  Integrator2/1 -> y/1, Sum3/2
  Sum3/1 -> Converter2/1
  Converter2/1 -> Integrator2/1
  u/1 -> Sum3/1

== system Powersystem_without_oscilloscopes/WindGenerator5/Machine-side converter ==
  u : Inport
  Converter2 : Gain  Gain=1/T
  Integrator2 : Integrator  InitialCondition=y0
  Sum3 : Sum  Inputs=|+-
  y : Outport
  wires:
  Integrator2/1 -> y/1, Sum3/2
  Sum3/1 -> Converter2/1
  Converter2/1 -> Integrator2/1
  u/1 -> Sum3/1

== system Powersystem_without_oscilloscopes/WindGenerator6/Grid-side converter ==
  u : Inport
  Converter2 : Gain  Gain=1/T
  Integrator2 : Integrator  InitialCondition=y0
  Sum3 : Sum  Inputs=|+-
  y : Outport
  wires:
  Integrator2/1 -> y/1, Sum3/2
  Sum3/1 -> Converter2/1
  Converter2/1 -> Integrator2/1
  u/1 -> Sum3/1

== system Powersystem_without_oscilloscopes/WindGenerator6/Machine-side converter ==
  u : Inport
  Converter2 : Gain  Gain=1/T
  Integrator2 : Integrator  InitialCondition=y0
  Sum3 : Sum  Inputs=|+-
  y : Outport
  wires:
  Integrator2/1 -> y/1, Sum3/2
  Sum3/1 -> Converter2/1
  Converter2/1 -> Integrator2/1
  u/1 -> Sum3/1

== system Powersystem_without_oscilloscopes/WindGenerator7/Grid-side converter ==
  u : Inport
  Converter2 : Gain  Gain=1/T
  Integrator2 : Integrator  InitialCondition=y0
  Sum3 : Sum  Inputs=|+-
  y : Outport
  wires:
  Integrator2/1 -> y/1, Sum3/2
  Sum3/1 -> Converter2/1
  Converter2/1 -> Integrator2/1
  u/1 -> Sum3/1

== system Powersystem_without_oscilloscopes/WindGenerator7/Machine-side converter ==
  u : Inport
  Converter2 : Gain  Gain=1/T
  Integrator2 : Integrator  InitialCondition=y0
  Sum3 : Sum  Inputs=|+-
  y : Outport
  wires:
  Integrator2/1 -> y/1, Sum3/2
  Sum3/1 -> Converter2/1
  Converter2/1 -> Integrator2/1
  u/1 -> Sum3/1

== system Powersystem_without_oscilloscopes/WindGenerator8/Grid-side converter ==
  u : Inport
  Converter2 : Gain  Gain=1/T
  Integrator2 : Integrator  InitialCondition=y0
  Sum3 : Sum  Inputs=|+-
  y : Outport
  wires:
  Integrator2/1 -> y/1, Sum3/2
  Sum3/1 -> Converter2/1
  Converter2/1 -> Integrator2/1
  u/1 -> Sum3/1

== system Powersystem_without_oscilloscopes/WindGenerator8/Machine-side converter ==
  u : Inport
  Converter2 : Gain  Gain=1/T
  Integrator2 : Integrator  InitialCondition=y0
  Sum3 : Sum  Inputs=|+-
  y : Outport
  wires:
  Integrator2/1 -> y/1, Sum3/2
  Sum3/1 -> Converter2/1
  Converter2/1 -> Integrator2/1
  u/1 -> Sum3/1
